simulink model "ship_Track_round"  (Simulink 10.3)
settings: Solver=ode45  StartTime=0.0  StopTime=1500  RelTol=1e-3  EnableMultiTasking=on
libraries: simulink x2
settings Model: Creator=Administrator  LastModifiedBy=1179956468
settings DataIOCC: LimitDataPoints=on
settings DebuggingCC: SolverPrmCheckMsg=warning
settings ConfigComp: CovSFcnEnable=off

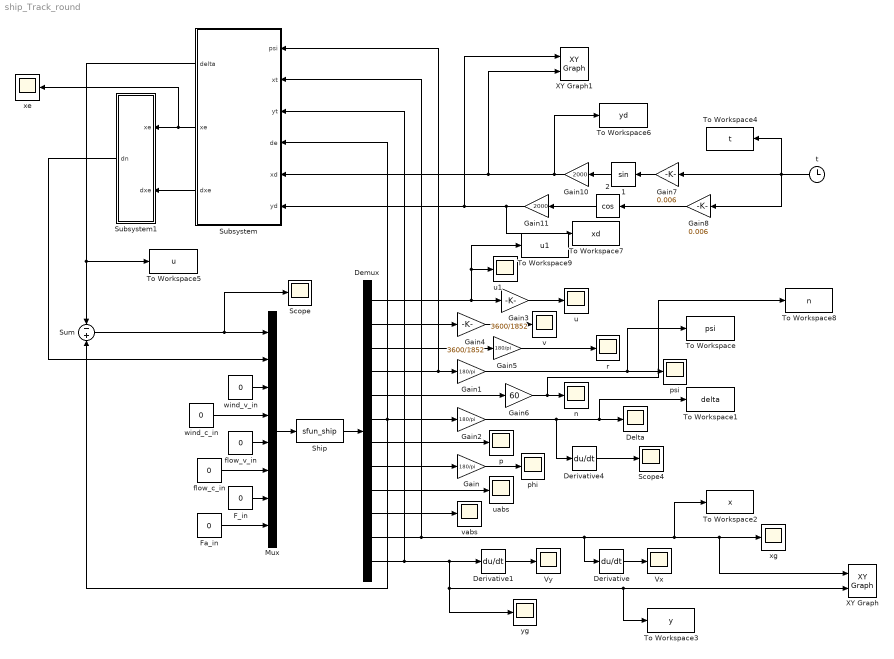
== system ship_Track_round ==
  "  1" : Trigonometry
  " 2" : Trigonometry  Operator=cos
  Delta : Scope
  Demux : Demux  Outputs=12
  Derivative : Derivative
  Derivative1 : Derivative
  Derivative4 : Derivative
  F_in : Constant  Value=0
  Fa_in : Constant  Value=0
  Gain{,1..2,5} (4 alike) : Gain  Gain=180/pi
  Gain10 : Gain  Gain=2000
  Gain11 : Gain  Gain=2000
  Gain3 : Gain  Gain=3600/1852
  Gain4 : Gain  Gain=3600/1852
  Gain6 : Gain  Gain=60
  Gain7 : Gain  Gain=0.006
  Gain8 : Gain  Gain=0.006
  Mux : Mux  Inputs=8
  Scope : Scope
  Scope4 : Scope
  Ship : S-Function  FunctionName=sfun_ship  SFunctionDeploymentMode=off  EnableBusSupport=off
  Subsystem : Subsystem
  Subsystem1 : Subsystem
  Sum : Sum  Inputs=-|+
  To Workspace : ToWorkspace  VariableName=psi  SampleTime=-1
  To Workspace1 : ToWorkspace  VariableName=delta  SampleTime=-1
  To Workspace2 : ToWorkspace  VariableName=x  SampleTime=-1
  To Workspace3 : ToWorkspace  VariableName=y  SampleTime=-1
  To Workspace4 : ToWorkspace  VariableName=t  SampleTime=-1
  To Workspace5 : ToWorkspace  VariableName=u  SampleTime=-1
  To Workspace6 : ToWorkspace  VariableName=yd  SampleTime=-1
  To Workspace7 : ToWorkspace  VariableName=xd  SampleTime=-1
  To Workspace8 : ToWorkspace  VariableName=n  SampleTime=-1
  To Workspace9 : ToWorkspace  VariableName=u1  SampleTime=-1
  "Vx " : Scope
  Vy : Scope
  XY Graph : simulink/Sinks/XY Graph  xmin=-3000  xmax=3000  ymin=-3000  ymax=3000  st=-1
  XY Graph1 : simulink/Sinks/XY Graph  xmin=-3000  xmax=3000  ymin=-3000  ymax=3000  st=-1
  flow_c_in : Constant  Value=0
  flow_v_in : Constant  Value=0
  n : Scope
  p : Scope
  phi : Scope
  psi : Scope
  r : Scope
  t : Clock
  u : Scope
  u1 : Scope
  uabs : Scope
  v : Scope
  vabs : Scope
  wind_c_in : Constant  Value=0
  wind_v_in : Constant  Value=0
  xe : Scope
  xg : Scope
  yg : Scope
  wires:
  Ship/1 -> Demux/1
  Demux/1 -> To Workspace9/1, u1/1, Gain3/1
  Demux/2 -> Gain4/1
  Demux/3 -> Gain5/1
  Demux/5 -> Gain6/1
  Demux/6 -> Gain2/1, Sum/2, Subsystem/4(de)
  Demux/7 -> p/1
  Demux/8 -> Gain/1
  Gain1/1 -> psi/1, To Workspace/1
  Gain/1 -> phi/1
  Gain3/1 -> u/1
  Gain4/1 -> v/1
  Gain5/1 -> r/1
  Gain6/1 -> To Workspace8/1, n/1
  Demux/9 -> uabs/1
  Demux/10 -> vabs/1
  Demux/12 -> Subsystem/3(yt), Derivative1/1, yg/1, To Workspace3/1, XY Graph/2
  Demux/11 -> Subsystem/2(xt), Derivative/1, To Workspace2/1, XY Graph/1, xg/1
  Derivative/1 -> "Vx "/1
  Derivative1/1 -> Vy/1
  wind_v_in/1 -> Mux/3
  wind_c_in/1 -> Mux/4
  flow_v_in/1 -> Mux/5
  F_in/1 -> Mux/7
  Fa_in/1 -> Mux/8
  flow_c_in/1 -> Mux/6
  Mux/1 -> Ship/1
  Derivative4/1 -> Scope4/1
  Subsystem/1(delta) -> Sum/1, To Workspace5/1
  Demux/4 -> Gain1/1, Subsystem/1(psi)
  Gain2/1 -> Derivative4/1, Delta/1, To Workspace1/1
  Sum/1 -> Mux/1, Scope/1
  "  1"/1 -> Gain10/1
  " 2"/1 -> Gain11/1
  t/1 -> Gain8/1, To Workspace4/1, Gain7/1
  Gain7/1 -> "  1"/1
  Gain8/1 -> " 2"/1
  Gain10/1 -> To Workspace6/1, XY Graph1/2, Subsystem/5(xd)
  Gain11/1 -> To Workspace7/1, XY Graph1/1, Subsystem/6(yd)
  Subsystem/2(xe) -> xe/1, Subsystem1/1(xe)
  Subsystem/3(dxe) -> Subsystem1/2(dxe)
  Subsystem1/1(dn) -> Mux/2

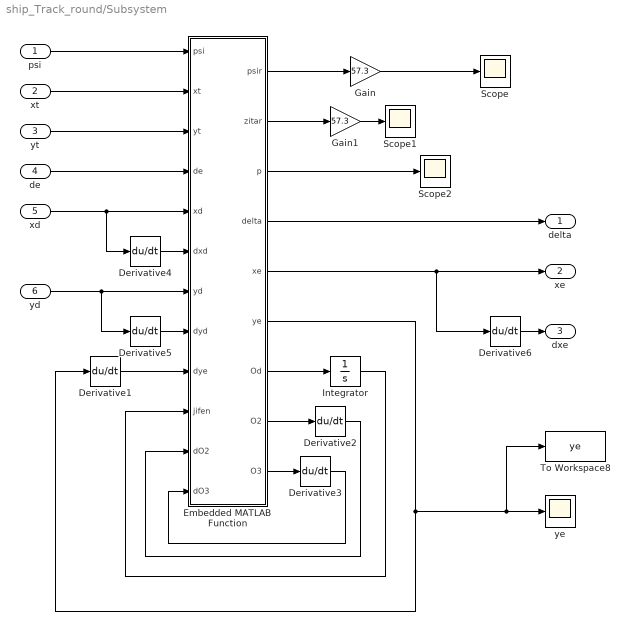
== system ship_Track_round/Subsystem ==
  psi : Inport
  xt : Inport  Port=2
  yt : Inport  Port=3
  de : Inport  Port=4
  xd : Inport  Port=5
  yd : Inport  Port=6
  Derivative{1..6} (6 alike) : Derivative
  Embedded MATLAB Function : MATLAB Function  TreatAsAtomicUnit=on
  Gain : Gain  Gain=57.3
  Gain1 : Gain  Gain=57.3
  Integrator : Integrator
  Scope : Scope
  Scope1 : Scope
  Scope2 : Scope
  To Workspace8 : ToWorkspace  VariableName=ye  SampleTime=-1
  ye : Scope
  delta : Outport
  xe : Outport  Port=2
  dxe : Outport  Port=3
  wires:
  Embedded MATLAB Function/9(O3) -> Derivative3/1
  Derivative3/1 -> Embedded MATLAB Function/12(dO3)
  Embedded MATLAB Function/8(O2) -> Derivative2/1
  Derivative2/1 -> Embedded MATLAB Function/11(dO2)
  Integrator/1 -> Embedded MATLAB Function/10(jifen)
  Embedded MATLAB Function/4(delta) -> delta/1
  Embedded MATLAB Function/7(Od) -> Integrator/1
  psi/1 -> Embedded MATLAB Function/1(psi)
  xt/1 -> Embedded MATLAB Function/2(xt)
  yt/1 -> Embedded MATLAB Function/3(yt)
  Derivative1/1 -> Embedded MATLAB Function/9(dye)
  Embedded MATLAB Function/6(ye) -> Derivative1/1, To Workspace8/1, ye/1
  de/1 -> Embedded MATLAB Function/4(de)
  xd/1 -> Derivative4/1, Embedded MATLAB Function/5(xd)
  yd/1 -> Derivative5/1, Embedded MATLAB Function/7(yd)
  Derivative4/1 -> Embedded MATLAB Function/6(dxd)
  Derivative5/1 -> Embedded MATLAB Function/8(dyd)
  Embedded MATLAB Function/5(xe) -> Derivative6/1, xe/1
  Derivative6/1 -> dxe/1
  Embedded MATLAB Function/1(psir) -> Gain/1
  Embedded MATLAB Function/2(zitar) -> Gain1/1
  Embedded MATLAB Function/3(p) -> Scope2/1
  Gain/1 -> Scope/1
  Gain1/1 -> Scope1/1

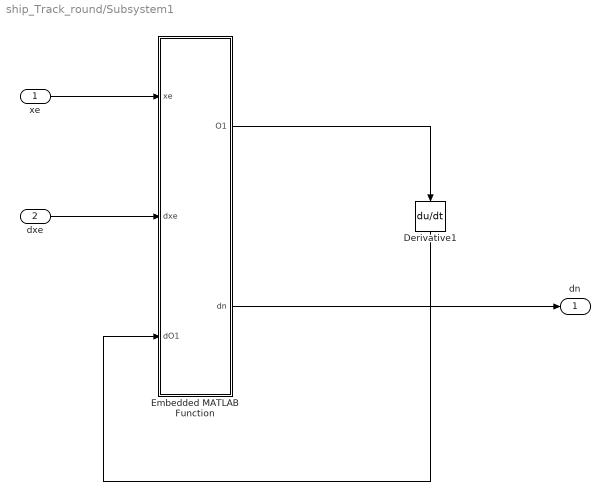
== system ship_Track_round/Subsystem1 ==
  xe : Inport
  dxe : Inport  Port=2
  Derivative1 : Derivative
  Embedded MATLAB Function : MATLAB Function  TreatAsAtomicUnit=on
  dn : Outport
  wires:
  xe/1 -> Embedded MATLAB Function/1(xe)
  Embedded MATLAB Function/1(O1) -> Derivative1/1
  Derivative1/1 -> Embedded MATLAB Function/3(dO1)
  dxe/1 -> Embedded MATLAB Function/2(dxe)
  Embedded MATLAB Function/2(dn) -> dn/1

== matlab function Subsystem1/Embedded MATLAB Function ==
  data: xe input double; dxe input double; dO1 input double; O1 output double; dn output double
function [O1,dn]=fcn(xe,dxe,dO1)
K11=4240;K12=3;K13=0.01;K14=0.0000005;K15=0.000006;K16=0;Tm=4;
%K11=3500;K12=3;K13=0.01;K14=0.0000005;K15=0.00006;K16=0;Tm=4;

O1=K11*tanh(K12*xe)+dxe;
O2=K13*tanh(K14*O1)+dO1;
dn=-K15*O2-K16*tanh(O2);
%nr=n+Tm*dn;

== matlab function Subsystem/Embedded MATLAB Function ==
  data: psir output double; zitar output double; p output double; psi input double; xt input double; yt input double; de input double; xd input double; dxd input double; yd input double; dyd input double; dye input double; delta output double; xe output double; ye output double; Od output double; O2 output double; O3 output double; jifen input double; dO2 input double; dO3 input double
function [psir,zitar,p,delta,xe,ye,Od,O2,O3] = fcn(psi,xt,yt,de,xd,dxd,yd,dyd,dye,jifen,dO2,dO3)

%K0=0.2;K1=0.005;K2=0.0004;K3=0.0000005;K4=3.4;K5=130;Te=2.5;
 K0=0.2;K1=0.005;K2=0.0003;K3=0.0000004;K4=3.4;K5=40;Te=2.5;
psir=atan2(dyd,dxd);
zitar=atan2((yt-yd),(xt-xd));%%%%%%%%%%%%%%%%%%%%%%
p=sqrt((xt-yd)^2+(yt-xd)^2);%%%%%%%%%%%%%%%%%%%%%%%%%%
xe=p*sin(zitar-psir);
ye=p*cos(zitar-psir);
% if(de>0)
%     psie=psi-psir-pi/2;
% else
%     psie=psi-psir+pi/2;
% end
 psie=psi-psir;

O1=K1*f(K0*ye)+dye;
Od=f(O1);
O2=psie+K2*jifen;
O3=K3*f(O2)+dO2;
O4=K4*f(O3)+dO3;
%delta=-K5*O4-K6*f(O4);%用舵机模型总是出错
delta=-Te*K5*O4;
 function mean=f(a)
  mean=tanh(a);
%  function mean=f(a)
%  if(a<0.1&&a>-0.1)
%      mean=a;
%  else
%      mean=coth(a)-1/a;
%  end
